simulink model "RateofWingEffects"  (R2024b)
settings: Solver=VariableStepAuto  StartTime=0.0  StopTime=10.0  RelTol=1e-3
undefined symbols (not defined in the file or in its folder): Aero
settings Model: Creator=Tyler  LastModifiedBy=Tyler

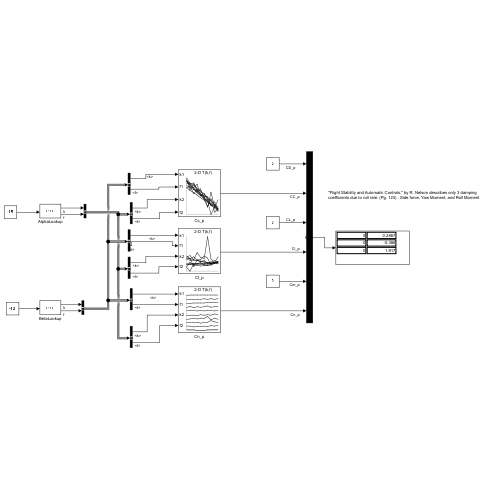
[thumbnail: Simulink's stored preview of the top-level diagram]
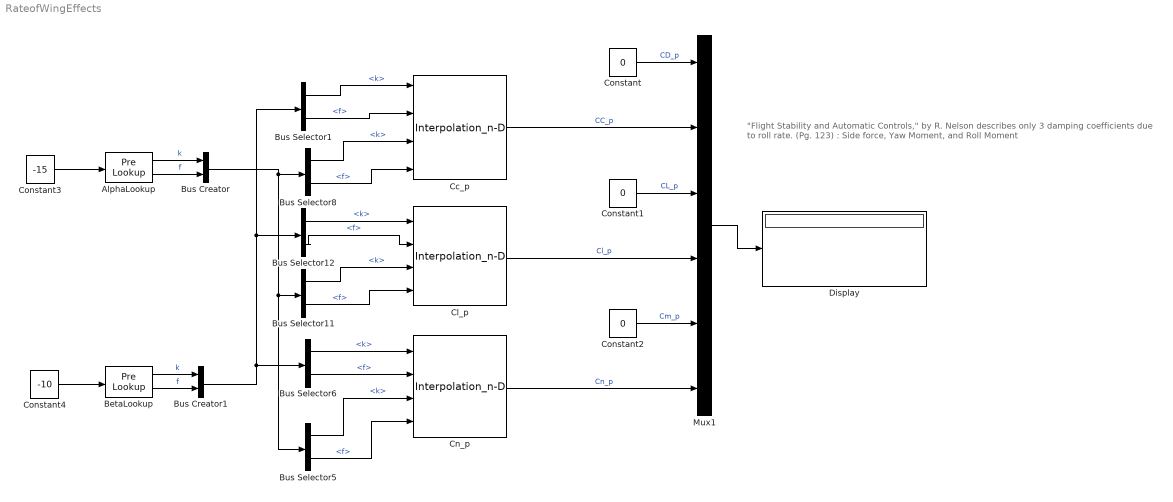
== system RateofWingEffects ==
  note: "Flight Stability and Automatic Controls," by R. Nelson describes only 3 damping coefficients due to roll rate. (Pg. 123) : Side force, Yaw Moment, and Roll Moment
  AlphaLookup : PreLookup  BreakpointsData=Aero.alpha_vec  BeginIndexSearchUsingPreviousIndexResult=on  ExtrapMethod=Linear
  BetaLookup : PreLookup  BreakpointsData=Aero.beta_vec  BeginIndexSearchUsingPreviousIndexResult=on  ExtrapMethod=Linear
  Bus Creator : BusCreator  Inputs=2
  Bus Creator1 : BusCreator  Inputs=2
  Bus Selector{1,5..6,8,11..12} (6 alike) : BusSelector  OutputSignals=k,f
  Cc_p : Interpolation_n-D  Table=Aero.Cc_p  ExtrapMethod=Clip  RemoveProtectionIndex=on  SaturateOnIntegerOverflow=on
  Cl_p : Interpolation_n-D  Table=Aero.Cl_p  ExtrapMethod=Clip  RemoveProtectionIndex=on  SaturateOnIntegerOverflow=on
  Cn_p : Interpolation_n-D  Table=Aero.Cn_p  ExtrapMethod=Clip  RemoveProtectionIndex=on  SaturateOnIntegerOverflow=on
  Constant : Constant  Value=0
  Constant1 : Constant  Value=0
  Constant2 : Constant  Value=0
  Constant3 : Constant  Value=-15
  Constant4 : Constant  Value=-10
  Display : Display
  Mux1 : Mux  Inputs=6
  wires:
  Bus Creator1/1 -> Bus Selector6/1, Bus Selector12/1, Bus Selector1/1
  Bus Selector12/2 -> Cl_p/2  "<f>"
  Cc_p/1 -> Mux1/2  "CC_p"
  Bus Selector5/2 -> Cn_p/4  "<f>"
  Constant/1 -> Mux1/1  "CD_p"
  Bus Creator/1 -> Bus Selector5/1, Bus Selector11/1, Bus Selector8/1
  Constant1/1 -> Mux1/3  "CL_p"
  Constant2/1 -> Mux1/5  "Cm_p"
  Bus Selector11/1 -> Cl_p/3  "<k>"
  Bus Selector8/2 -> Cc_p/4  "<f>"
  Cn_p/1 -> Mux1/6  "Cn_p"
  Bus Selector1/1 -> Cc_p/1  "<k>"
  Bus Selector8/1 -> Cc_p/3  "<k>"
  Mux1/1 -> Display/1
  Bus Selector5/1 -> Cn_p/3  "<k>"
  Bus Selector11/2 -> Cl_p/4  "<f>"
  Bus Selector6/2 -> Cn_p/2  "<f>"
  Bus Selector1/2 -> Cc_p/2  "<f>"
  Bus Selector12/1 -> Cl_p/1  "<k>"
  Bus Selector6/1 -> Cn_p/1  "<k>"
  Cl_p/1 -> Mux1/4  "Cl_p"
  Constant4/1 -> BetaLookup/1
  Constant3/1 -> AlphaLookup/1
  AlphaLookup/2 -> Bus Creator/2  "f"
  AlphaLookup/1 -> Bus Creator/1  "k"
  BetaLookup/2 -> Bus Creator1/2  "f"
  BetaLookup/1 -> Bus Creator1/1  "k"
